simulink model "inverter_control_average_model"  (Simulink 8.5)
settings: Solver=ode23s  StartTime=0.0  StopTime=0.1  RelTol=1e-3
values from neighbouring files (symbols this model uses):
  f_grid = 50    [inverter_settings.m]
  Kp = 2    [inverter_settings.m]
  L_f = 2e-3    (= 0.002)    [inverter_settings.m]
  R_f = 10e-3    (= 0.01)    [inverter_settings.m]
  Ti = 10e-3    (= 0.01)    [inverter_settings.m]
  V_dc = 700    [inverter_settings.m]
  V_grid = 230    [inverter_settings.m]
undefined symbols (not defined in the file or in its folder): j
libraries: powerlib x20, powerlib_meascontrol x2
settings Model: Creator=Pierre  LastModifiedBy=Pierre
settings DataIOCC: SignalLoggingSaveFormat=Dataset
settings OptimizationCC: ExpressionDepthLimit=128
settings DebuggingCC: UnderspecifiedInitializationDetection=Simplified  MergeDetectMultiDrivingBlocksExec=error  FcnCallInpInsideContextMsg=EnableAllAsError  StateNameClashWarn=none
settings GRTTargetCC: CombineOutputUpdateFcns=on  GRTInterface=off

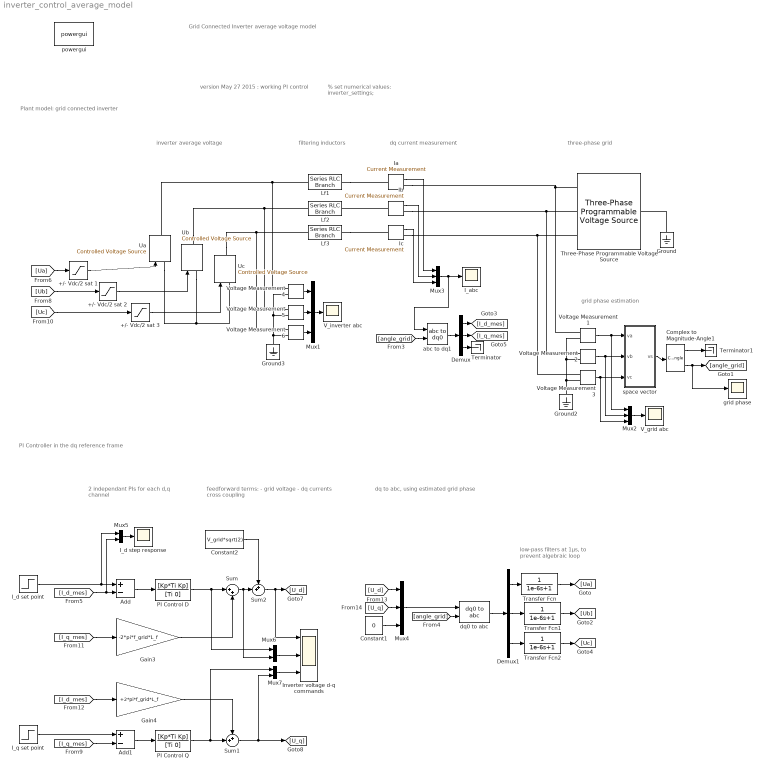
== system inverter_control_average_model ==
  note: feedforward terms:
      | - grid voltage
      | - dq currents cross coupling
  note: PI Controller
      | in the dq reference frame
  note: % set numerical values:
      | inverter_settings;
  note: version May 27 2015 : working PI control
  note: Grid Connected Inverter
      | average voltage model
  note: 2 independant PIs
      | for each d,q channel
  note: dq to abc,
      | using estimated grid phase
  note: low-pass filters at 1µs,
      | to prevent algebraic loop
  note: inverter average voltage
  note: Plant model: grid connected inverter
  note: filtering inductors
  note: three-phase grid
  note: dq current measurement
  note: grid phase estimation
  +/- Vdc/2 sat 1 : Saturate  UpperLimit=V_dc/2  LowerLimit=-V_dc/2
  +/- Vdc/2 sat 2 : Saturate  UpperLimit=V_dc/2  LowerLimit=-V_dc/2
  +/- Vdc/2 sat 3 : Saturate  UpperLimit=V_dc/2  LowerLimit=-V_dc/2
  Add : Sum  Inputs=+-
  Add1 : Sum  Inputs=+-
  Complex to Magnitude-Angle1 : ComplexToMagnitudeAngle
  Constant1 : Constant  Value=0
  Constant2 : Constant  Value=V_grid*sqrt(2)
  Demux : Demux  Outputs=3
  Demux1 : Demux  Outputs=3
  Gain3 : Gain  Gain=-2*pi*f_grid*L_f
  Gain4 : Gain  Gain=+2*pi*f_grid*L_f
  Ground : powerlib/Elements/Ground  LConnTagsString=a
  Ground2 : powerlib/Elements/Ground  LConnTagsString=a
  Ground3 : powerlib/Elements/Ground  LConnTagsString=a
  I_abc : Scope
      settings: TimeRange=2  YMin=0  YMax=12
  I_d set point : Step  Time=0.03  After=10  SampleTime=0
  I_d step response : Scope
      settings: TimeRange=2  YMin=-15  YMax=15  SaveName=ScopeData7
  I_q set point : Step  Time=0.01  After=0  SampleTime=0
  Ia : powerlib/Measurements/Current Measurement  PhasorSimulation=off  OutputType=Complex  PSBequivalent=0
  Ib : powerlib/Measurements/Current Measurement  PhasorSimulation=off  OutputType=Complex  PSBequivalent=0
  Ic : powerlib/Measurements/Current Measurement  PhasorSimulation=off  OutputType=Complex  PSBequivalent=0
  Inverter voltage d-q commands : Scope  NumInputPorts=3
      settings: TimeRange=2  YMin=0~-5~-5  YMax=12~5~5  SaveName=ScopeData6
  Lf1 : powerlib/Elements/Series RLC Branch  LConnTagsString=__new0  RConnTagsString=__new0  BranchType=RL  Resistance=R_f  Inductance=L_f  SetiL0=off  InitialCurrent=0  Capacitance=1e-6  Setx0=off  InitialVoltage=0  Measurements=None
  Lf2 : powerlib/Elements/Series RLC Branch  LConnTagsString=__new0  RConnTagsString=__new0  BranchType=RL  Resistance=R_f  Inductance=L_f  SetiL0=on  InitialCurrent=0  Capacitance=1e-6  Setx0=off  InitialVoltage=0  Measurements=None
  Lf3 : powerlib/Elements/Series RLC Branch  LConnTagsString=__new0  RConnTagsString=__new0  BranchType=RL  Resistance=R_f  Inductance=L_f  SetiL0=on  InitialCurrent=0  Capacitance=1e-6  Setx0=off  InitialVoltage=0  Measurements=None
  Mux{1..4} (4 alike) : Mux  Inputs=3
  Mux5 : Mux  Inputs=2
  Mux6 : Mux  Inputs=2
  Mux7 : Mux  Inputs=2
  PI Control D : TransferFcn  Numerator=[Kp*Ti Kp]  Denominator=[Ti 0]
  PI Control Q : TransferFcn  Numerator=[Kp*Ti Kp]  Denominator=[Ti 0]
  Sum : Sum  Inputs=|++
  Sum1 : Sum  Inputs=++|
  Sum2 : Sum  Inputs=++|
  Terminator : Terminator
  Terminator1 : Terminator
  Three-Phase Programmable Voltage Source : powerlib/Electrical Sources/Three-Phase Programmable Voltage Source  PositiveSequence="[V_grid*sqrt(3)  0 50]"  VariationEntity=None  VariationType=Table of time-amplitude pairs  VariationTypeAlt=Step  VariationStep=0.5  VariationRate=10  VariationMagnitude=0.3  VariationFrequency=2  VariationTiming=[1 2]  VariationPhaseA=off  Amplitudes=[1 0.8 1.2 1.0]  TimeValues=[0 0.1 0.15 0.2]  HarmonicGeneration=off  HarmonicA=[3 0.2 -25 0]  HarmonicB=[2 0.15 35 2]  Timing="[0.05  3]"  BusType=swing  Pref=0  Qref=0  Qmin=-inf  Qmax=inf
  Transfer Fcn : TransferFcn  Denominator=[1e-6 1]
  Transfer Fcn1 : TransferFcn  Denominator=[1e-6 1]
  Transfer Fcn2 : TransferFcn  Denominator=[1e-6 1]
  Ua : powerlib/Electrical Sources/Controlled Voltage Source  Initialize=off  Source_Type=AC  Amplitude=0  Phase=0  Frequency=0  Measurements=None
  Ub : powerlib/Electrical Sources/Controlled Voltage Source  Initialize=off  Source_Type=AC  Amplitude=0  Phase=0  Frequency=0  Measurements=None
  Uc : powerlib/Electrical Sources/Controlled Voltage Source  Initialize=off  Source_Type=AC  Amplitude=0  Phase=0  Frequency=0  Measurements=None
  V_grid abc : Scope
      settings: TimeRange=2  YMin=0  YMax=12  SaveName=ScopeData2
  V_inverter abc : Scope
      settings: TimeRange=2  YMin=0  YMax=12
  Voltage Measurement{1..6} (6 alike) : powerlib/Measurements/Voltage Measurement  PhasorSimulation=off  OutputType=Complex  PSBequivalent=0
  abc to dq1 : powerlib_meascontrol/Transformations/abc to dq0  Alignment=Aligned with phase A axis
  dq0 to abc : powerlib_meascontrol/Transformations/dq0 to abc  Alignment=Aligned with phase A axis
  grid phase : Scope
      settings: TimeRange=2  YMin=0  YMax=12  SaveName=ScopeData3
  powergui : powerlib/powergui  Priority=1  SimulationMode=Continuous  SolverType=Tustin/Backward Euler (TBE)  SampleTime=50e-6  frequency=60  SPID=on  DisableSnubberDevices=on  DisableRonSwitches=on  DisableVfSwitches=on  SwTol=0  DisplayEquations=off  Interpol=off  methode=off  Ts=100  FunctionMessages=off  echomessages=off  HookPort=off  EnableUseOfTLC=off  x0status=blocks  frequencyindice=50  Pbase=100e6  ErrMax=1e-4  Iterations=50  UnitsV=kV  UnitsW=MW  buscounter=0  RestoreLinks=warning  ResistiveCurrentMeasurement=off  Frange=[0:2:500]  Ylog=off  Xlog=on  ShowGrid=off  save=off  variable=ZData  structure=0  ZoomFFT=off  StartTime=0.0  cycles=1  DisplayStyle=1  fundamental=60  FreqAxis=off  MaxFrequency=1000  frequencyindicesteady=1  RmsSteady=1  display=off
  space vector : Subsystem
  wires:
  Mux1/1 -> V_inverter abc/1
  Voltage Measurement1/1 -> Mux2/1, space vector/1(va)
  Voltage Measurement2/1 -> Mux2/2, space vector/2(vb)
  Voltage Measurement3/1 -> space vector/3(vc), Mux2/3
  space vector/1(vs) -> Complex to Magnitude-Angle1/1
  Mux2/1 -> V_grid abc/1
  [Ua] -> +/- Vdc/2 sat 1/1
  [Ub] -> +/- Vdc/2 sat 2/1
  [Uc] -> +/- Vdc/2 sat 3/1
  Mux3/1 -> I_abc/1, abc to dq1/1
  Ia/1 -> Mux3/1
  Ib/1 -> Mux3/2
  Ic/1 -> Mux3/3
  Voltage Measurement4/1 -> Mux1/1
  Voltage Measurement5/1 -> Mux1/2
  Voltage Measurement6/1 -> Mux1/3
  Complex to Magnitude-Angle1/2 -> [angle_grid], grid phase/1
  [angle_grid] -> abc to dq1/2
  abc to dq1/1 -> Demux/1
  Demux/1 -> [I_d_mes]
  Demux/2 -> [I_q_mes]
  Demux/3 -> Terminator/1
  [angle_grid] -> dq0 to abc/2
  [I_d_mes] -> Mux5/2, Add/2
  I_d set point/1 -> Mux5/1, Add/1
  Add/1 -> PI Control D/1
  Mux4/1 -> dq0 to abc/1
  Demux1/1 -> Transfer Fcn/1
  [I_q_mes] -> Add1/2
  I_q set point/1 -> Add1/1
  Add1/1 -> PI Control Q/1
  Complex to Magnitude-Angle1/1 -> Terminator1/1
  Demux1/2 -> Transfer Fcn1/1
  Demux1/3 -> Transfer Fcn2/1
  Gain4/1 -> Sum1/1
  PI Control Q/1 -> Mux7/1, Sum1/2
  dq0 to abc/1 -> Demux1/1
  Sum/1 -> Mux6/2, Sum2/2
  Mux5/1 -> I_d step response/1
  Sum2/1 -> Inverter voltage d-q commands/1, [U_d]
  Sum1/1 -> Mux7/2, [U_q]
  Gain3/1 -> Sum/2
  PI Control D/1 -> Mux6/1, Sum/1
  [U_d] -> Mux4/1
  [U_q] -> Mux4/2
  Constant1/1 -> Mux4/3
  Mux6/1 -> Inverter voltage d-q commands/2
  Mux7/1 -> Inverter voltage d-q commands/3
  Transfer Fcn/1 -> [Ua]
  Transfer Fcn1/1 -> [Ub]
  Transfer Fcn2/1 -> [Uc]
  +/- Vdc/2 sat 1/1 -> Ua/1
  +/- Vdc/2 sat 2/1 -> Ub/1
  +/- Vdc/2 sat 3/1 -> Uc/1
  [I_q_mes] -> Gain3/1
  [I_d_mes] -> Gain4/1
  Constant2/1 -> Sum2/1
  connections:
  Voltage Measurement2/LConn1 -- Three-Phase Programmable Voltage Source/RConn2 -- Ib/RConn1
  Voltage Measurement3/LConn1 -- Ic/RConn1 -- Three-Phase Programmable Voltage Source/RConn3
  Voltage Measurement1/LConn1 -- Ia/RConn1 -- Three-Phase Programmable Voltage Source/RConn1
  Ground/LConn1 -- Three-Phase Programmable Voltage Source/LConn1
  Ua/RConn1 -- Voltage Measurement4/LConn1 -- Lf1/LConn1
  Ub/LConn1 -- Uc/LConn1 -- Ua/LConn1
  Ground2/LConn1 -- Voltage Measurement3/LConn2 -- Voltage Measurement2/LConn2 -- Voltage Measurement1/LConn2
  Uc/RConn1 -- Lf3/LConn1 -- Voltage Measurement6/LConn1
  Ub/RConn1 -- Lf2/LConn1 -- Voltage Measurement5/LConn1
  Lf1/RConn1 -- Ia/LConn1
  Ib/LConn1 -- Lf2/RConn1
  Lf3/RConn1 -- Ic/LConn1
  Voltage Measurement5/LConn2 -- Voltage Measurement4/LConn2 -- Voltage Measurement6/LConn2 -- Ground3/LConn1

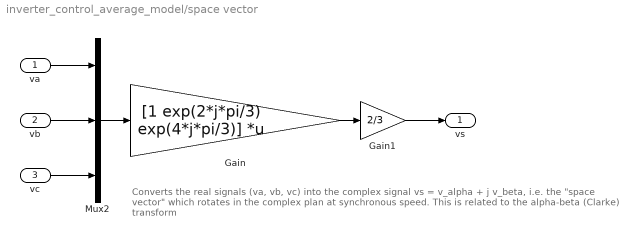
== system inverter_control_average_model/space vector ==
  note: Converts the real signals (va, vb, vc)
      | into the complex signal vs = v_alpha + j v_beta, i.e. the "space vector" which rotates in the complex plan at synchronous speed.
      | This is related to the alpha-beta (Clarke) transform
  va : Inport
  vb : Inport  Port=2
  vc : Inport  Port=3
  Gain : Gain  Gain=[1 exp(2*j*pi/3) exp(4*j*pi/3)]  Multiplication=Matrix(K*u) (u vector)
  Gain1 : Gain  Gain=2/3
  Mux2 : Mux  Inputs=3
  vs : Outport
  wires:
  Mux2/1 -> Gain/1
  vb/1 -> Mux2/2
  Gain1/1 -> vs/1
  va/1 -> Mux2/1
  Gain/1 -> Gain1/1
  vc/1 -> Mux2/3
